simulink model "Simulate_Cart_Inverted_Pend_r2018a"  (R2020a)
settings: Solver=VariableStepAuto  StartTime=0.0  StopTime=10  RelTol=1e-3
undefined symbols (not defined in the file or in its folder): drawPendulum
libraries: simulink_extras x1
settings Model: Creator=7247239  LastModifiedBy=jem2
settings DataIOCC: LimitDataPoints=on  SaveOutput=off  SaveTime=off  ReturnWorkspaceOutputs=off
settings OptimizationCC: BlockReduction=off  BooleanDataType=off  LifeSpan=inf
settings DebuggingCC: SaveWithParameterizedLinksMsg=none  UnderspecifiedInitializationDetection=Classic  MergeDetectMultiDrivingBlocksExec=none  SignalResolutionControl=TryResolveAllWithWarning  AllowSymbolicDim=off  SFUnexpectedBacktrackingDiag=warning  SFNoUnconditionalDefaultTransitionDiag=warning  SFExecutionAtInitializationDiag=none  ArithmeticOperatorsInVariantConditions=warning
settings HardwareCC: TargetUnknown=on
settings SFSimCC: SimUseLocalCustomCode=off  CustomCodeUndefinedFunction=UseInterfaceOnly
settings RTWCC: RTWUseLocalCustomCode=off
settings CodeAppCC: StateflowObjectComments=on
settings GRTTargetCC: TargetLangStandard=C89/C90 (ANSI)
settings ConfigComp: CovMetricSettings=dw  CovHtmlReporting=on  CovSaveCumulativeToWorkspaceVar=on  CovSaveSingleToWorkspaceVar=on  CovExternalEMLEnable=off

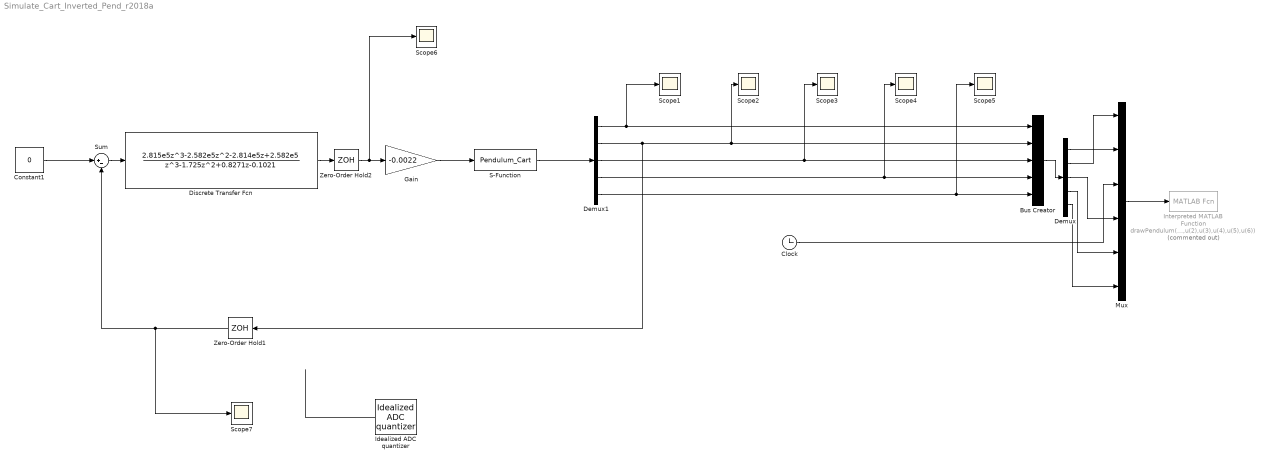
== system Simulate_Cart_Inverted_Pend_r2018a ==
  Bus Creator : BusCreator  Inputs=5
  Clock : Clock
  Constant1 : Constant  Value=0
  Demux : Demux  Outputs=5
  Demux1 : Demux  Outputs=5
  Discrete Transfer Fcn : DiscreteTransferFcn  Numerator=[2.815e5 -2.582e5 -2.814e5 2.582e5]  Denominator=[1 -1.725 0.8271 -0.1021]
  Gain : Gain  Gain=-0.0022
  Idealized ADC quantizer : simulink_extras/Additional Discrete/Idealized ADC quantizer  NumberOfConverterBits=12  Vmin=0  Vmax=5  OutputDataType=int16  OutputNegativeValues=off
  Interpreted MATLAB Function : MATLABFcn  Commented=on  MATLABFcn=drawPendulum(u(1),u(2),u(3),u(4),u(5),u(6))  OutputDimensions=0
  Mux : Mux  Inputs=6
  S-Function : S-Function  FunctionName=Pendulum_Cart  Parameters=0.9540, -9.81, 1.2446, 0.0760, 0, w, h  SFunctionDeploymentMode=off  EnableBusSupport=off
      mask init:
      | g=9.81;
      | L=2;
      | b=0;
      | m=1000;
      | M=1;
      | w=.5;
      | h=.2;
  Scope{1..7} (7 alike) : Scope
  Sum : Sum  Inputs=|+-
  Zero-Order Hold1 : ZeroOrderHold  SampleTime=-1
  Zero-Order Hold2 : ZeroOrderHold  SampleTime=0.01
  wires:
  Clock/1 -> Mux/3
  Constant1/1 -> Sum/1
  Demux/1 -> Mux/1
  Demux/2 -> Mux/2
  Demux/3 -> Mux/4
  Demux/4 -> Mux/5
  Demux/5 -> Mux/6
  S-Function/1 -> Demux1/1
  Demux1/2 -> Zero-Order Hold1/1, Scope2/1, Bus Creator/2
  Bus Creator/1 -> Demux/1
  Demux1/1 -> Scope1/1, Bus Creator/1
  Demux1/3 -> Scope3/1, Bus Creator/3
  Demux1/4 -> Scope4/1, Bus Creator/4
  Demux1/5 -> Scope5/1, Bus Creator/5
  Mux/1 -> Interpreted MATLAB Function/1
  Gain/1 -> S-Function/1
  Idealized ADC quantizer/1 -> ?
  Zero-Order Hold1/1 -> Scope7/1, Sum/2
  Zero-Order Hold2/1 -> Scope6/1, Gain/1
  Discrete Transfer Fcn/1 -> Zero-Order Hold2/1
  Sum/1 -> Discrete Transfer Fcn/1
